simulink model "MPCcontrolledSpacecraft_plant_gnss_kalman_decision"  (R2025b)
settings: Solver=ode113  StartTime=0.0  StopTime=tf  FixedStep=1*60*60  RelTol=1e-8  AbsTol=1e-8
InitFcn:
  | %--- AUTO-INSERTED BY setup_instrument_decision (do not edit by hand)
  | if exist('load_gnss_quality_signals', 'file') == 2
  |     load_gnss_quality_signals('cov_perturb_POS_s6a_Y24D011_fixed.dat');
  | end
  | %--- END AUTO-INSERTED
values from neighbouring files (symbols this model uses):
  area = 15    [Script_Concurso_Spacecraft_batch.m]
  gnss_sample_time = gnssSensor.sample_time    [Script_Concurso_Spacecraft_batch.m]
  h = norm(h_vec)    [Script_Concurso_Spacecraft_batch.m]
  initMass = m_sat    (= 10000)    [Script_Concurso_Spacecraft_batch.m]
  lamda_init = 1    [Script_Concurso_Spacecraft_batch.m]
  m = 3    [Script_Concurso_Spacecraft_batch.m]
  ref = 1.3    [Script_Concurso_Spacecraft_batch.m]
  s = [sigma_x,sigma_x,sigma_x,sigma_v,sigma_v,sigma_v]    [Script_Concurso_Spacecraft_batch.m]
  Ts = 1    [Script_Concurso_Spacecraft_batch.m]
  var_alt = sigma_alt^2    (= 2500)    [Script_Concurso_Spacecraft_batch.m]
  var_IMU = 0.01    [Script_Concurso_Spacecraft_batch.m]
  var_pos = sigma_pos^2    (= 10000)    [Script_Concurso_Spacecraft_batch.m]
undefined symbols (not defined in the file or in its folder): endDate, thrustingThreshold
libraries: simulink x6, vrlib x2, sharedTrackingLibrary x1, aerolibsatdyn x1, aerolibutil x1
settings Model: SimulationMode=accelerator  Creator=benit  LastModifiedBy=benit
settings DebuggingCC: UnderSpecifiedDimensionMsg=warning

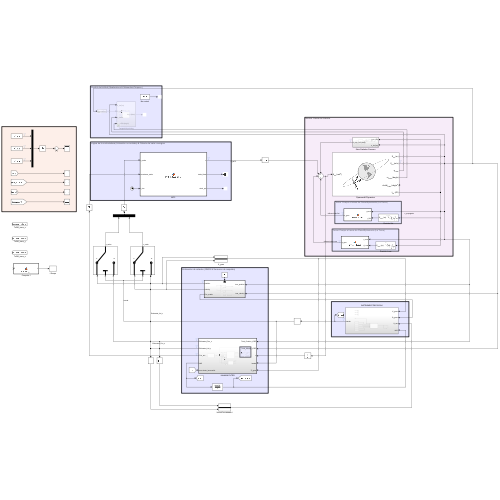
[thumbnail: Simulink's stored preview of the top-level diagram]
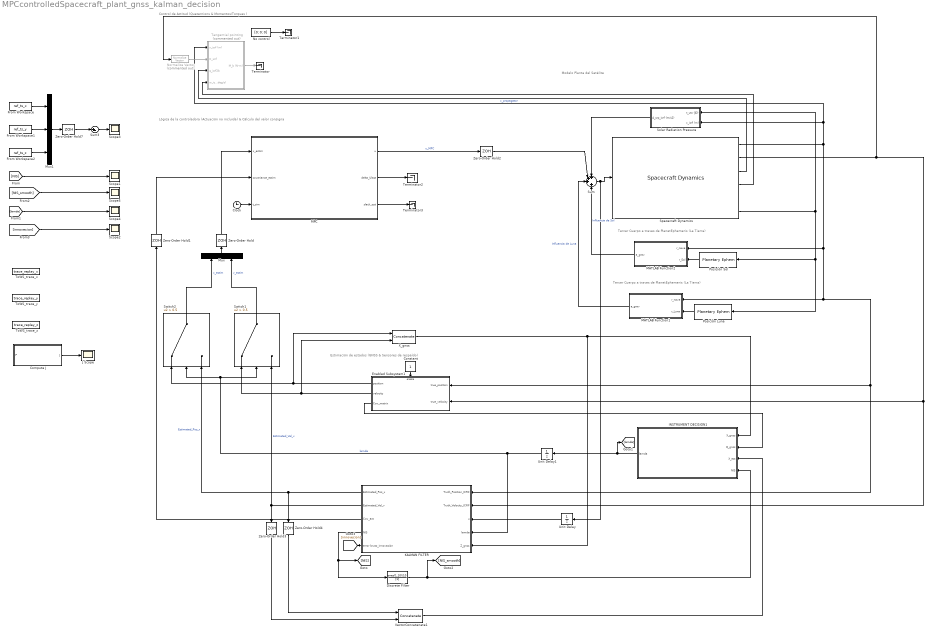
== system MPCcontrolledSpacecraft_plant_gnss_kalman_decision ==
  note: Control de Actitud (Quaternions & Momentos/Torques )
  note: Lógica de la controladora (Actuación no incluida) & Cálculo del valor consigna
  note: Estimación de estados (GNSS & Sensores de respaldo)
  note: Modelo Planta del Satélite
  note: Tercer Cuerpo a traves de PlanetEphemeris (La Tierra)
  note: Tercer Cuerpo a traves de PlanetEphemeris (La Tierra)
  Clock : Clock
      settings: Decimation=h
  Compute J : MATLAB Function  TreatAsAtomicUnit=on
  Constant : Constant
  Discrete Filter : DiscreteFilter  Numerator=ones(1,10)/10  Denominator=[1]
  Enabled Subsystem1 : Subsystem  Description=|  TreatAsAtomicUnit=on
      | "GNSS ON"
      | 
      | Aquí va a ir las medidas del vector de estados utilizando GNSS. 
      | 
      | Se tendrá que añadir todo el sistema de ruido blanco del sensor, así como la regresión
      | por medio de mínimos cuadrados (WLSQ)
  From Workspace : FromWorkspace  VariableName=ref_ts_x  SampleTime=1
  From Workspace1 : FromWorkspace  VariableName=ref_ts_y  SampleTime=1
  From Workspace2 : FromWorkspace  VariableName=ref_ts_z  SampleTime=1
  INSTRUMENT DECISION1 : Subsystem
  J Scope : Scope
      settings: ActiveDisplayYMinimum=-61.078405392126143  ActiveDisplayYMaximum=582.31960931045694
  KALMAN FILTER : Subsystem  Description=|  TreatAsAtomicUnit=on
      | "GNSS OFF"
      | 
      | Aquí va a ir las medidas del vector de estados utilizando Backup Sensor. 
      | 
      | Se tendrá que añadir todo el sistema de ruido blanco de los sensor de respaldo, 
      | así como el Filtro de Kalman y la estadística que permita mezclar las distintas medidas 
      | de distinta procedencia.
  MATLAB Function1 : MATLAB Function  TreatAsAtomicUnit=on
  MATLAB Function2 : MATLAB Function  TreatAsAtomicUnit=on
  MPC : MATLAB Function  TreatAsAtomicUnit=on  SystemSampleTime=h
  Mux : Mux  Inputs=2
  Mux1 : Mux  Inputs=3
  No control : Constant  Value=[0; 0; 0]
  Normalize Vector : vrlib/Utilities/Normalize Vector  Commented=on  maxzero=0
  Posición Luna : PlanetaryEphem  units=m,m/s  center=Sun  startDate=startDate2  endDate=endDate*1.02  outputVelocity=off
  Posición Sol : PlanetaryEphem  units=m,m/s  target=Sun  startDate=startDate2  endDate=endDate*1.02  outputVelocity=off
  Scope{1..5} (5 alike) : Scope
      Scope1 settings: ActiveDisplayYMinimum=-148.75157681735678  ActiveDisplayYMaximum=1338.765518425161
      Scope2 settings: ActiveDisplayYMinimum=-421.91395094944164  ActiveDisplayYMaximum=389.67502541979775  DataLoggingVariableName=ScopeData9
      Scope3 settings: ActiveDisplayYMinimum=-16012.819311832352  ActiveDisplayYMaximum=11977.80759284162  DataLoggingVariableName=ScopeData5
      Scope4 settings: ActiveDisplayYMinimum=-0.12499999999999997  ActiveDisplayYMaximum=1.125  DataLoggingVariableName=ScopeData2
      Scope5 settings: ActiveDisplayYMinimum=-29.897403423774861  ActiveDisplayYMaximum=269.07860039987031  DataLoggingVariableName=ScopeData6
  Solar Radiation Pressure : Subsystem
  Spacecraft Dynamics : SpacecraftDynamics  forcesIn=off  momentsIn=off  accelIn=on  startDate=start_date  mass=m_sat  semiMajorAxis=a  eccentricity=ecc  inclination=inc  raan=RAAN  argPeriapsis=w  trueAnomaly=theta  outputAngAccel=on  shDegree=2  ephemerisStartDate=start_date  ephemerisEndDate=start_date
  Sum : Sum  Inputs=+++|+
  Sum3 : Sum  Inputs=|+-
  Switch1 : Switch  Criteria=u2 > Threshold  Threshold=0.5  SaturateOnIntegerOverflow=off  InputSameDT=off
  Switch2 : Switch  Criteria=u2 > Threshold  Threshold=0.5  SaturateOnIntegerOverflow=off  InputSameDT=off
  Tangential pointing : Subsystem  Commented=on
  Terminator{,1..3} (4 alike) : Terminator
  ToWS_trace_x : ToWorkspace  VariableName=trace_replay_x  SampleTime=-1
  ToWS_trace_y : ToWorkspace  VariableName=trace_replay_y  SampleTime=-1
  ToWS_trace_z : ToWorkspace  VariableName=trace_replay_z  SampleTime=-1
  Unit Delay : UnitDelay  InitialCondition=[0; 0; 0]  SampleTime=Ts  HasFrameUpgradeWarning=on
  Unit Delay1 : UnitDelay  InitialCondition=lamda_init  SampleTime=Ts  HasFrameUpgradeWarning=on
  VectorConcatenate1 : Concatenate
  X_gnss : Concatenate
  Zero-Order Hold{,1..4,7} (6 alike) : ZeroOrderHold  SampleTime=h
  wires:
  Spacecraft Dynamics/1 -> Tangential pointing/1(x_icrf (m)), Solar Radiation Pressure/2(x_icrf (m)), Enabled Subsystem1/1(true_position), KALMAN FILTER/1(Truth_Position_ICRF), MATLAB Function1/1(r_nave), MATLAB Function2/1(r_nave)  "x_propagator"
  Spacecraft Dynamics/6 -> Solar Radiation Pressure/1(t_utc (JD)), Posición Luna/1, Posición Sol/1
  Posición Sol/1 -> MATLAB Function2/2(r_Sol)
  Posición Luna/1 -> MATLAB Function1/2(r_Luna)
  Unit Delay1/1 -> Switch2/2, Switch1/2, KALMAN FILTER/4(lamda)  "lamda"
  Spacecraft Dynamics/2 -> KALMAN FILTER/2(Truth_Velocity_ICRF), Enabled Subsystem1/2(true_velocity), Normalize Vector/1
  Enabled Subsystem1/1(position) -> Switch2/1, X_gnss/1
  KALMAN FILTER/1(Estimated_Pos_x) -> Switch2/3, Zero-Order Hold4/1  "Estimated_Pos_x"
  Spacecraft Dynamics/4 -> Tangential pointing/4(w_icrf2b (deg/s))
  Spacecraft Dynamics/3 -> Tangential pointing/3(q_icrf2b)
  Normalize Vector/1 -> Tangential pointing/2(C_icrf)
  Tangential pointing/1(M_b (N-m)) -> Terminator/1
  No control/1 -> Terminator1/1
  Enabled Subsystem1/2(velocity) -> Switch1/1, X_gnss/2
  KALMAN FILTER/2(Estimated_Vel_v) -> Switch1/3, Zero-Order Hold3/1  "Estimated_Vel_v"
  Solar Radiation Pressure/1(A_srp_icrf (m/s2)) -> Sum/1
  MATLAB Function2/1(a_grav) -> Sum/4  "Influencia de Sol"
  MATLAB Function1/1(a_grav) -> Sum/3  "Influencia de Luna"
  Sum/1 -> Spacecraft Dynamics/1, Unit Delay/1
  KALMAN FILTER/3(Cov_act) -> Zero-Order Hold1/1
  Unit Delay/1 -> KALMAN FILTER/3(u)
  Mux/1 -> Zero-Order Hold/1
  MPC/1(u) -> Zero-Order Hold2/1  "u_MPC"
  MPC/2(delta_Ulast) -> Terminator2/1
  MPC/3(slack_opt) -> Terminator3/1
  Zero-Order Hold/1 -> MPC/1(x_estim)
  Zero-Order Hold1/1 -> MPC/2(covariance_estim)
  Zero-Order Hold2/1 -> Sum/2
  Clock/1 -> MPC/3(t_sim)
  X_gnss/1 -> KALMAN FILTER/5(Z_gnss), INSTRUMENT DECISION1/1(X_gnss)
  Enabled Subsystem1/3(Cov_matrix) -> INSTRUMENT DECISION1/2(Q_gnss)
  VectorConcatenate1/1 -> INSTRUMENT DECISION1/3(X_est)
  Zero-Order Hold3/1 -> VectorConcatenate1/2
  Zero-Order Hold4/1 -> VectorConcatenate1/1
  Switch2/1 -> Mux/1  "x_estim"
  Switch1/1 -> Mux/2  "v_estim"
  Constant/1 -> Enabled Subsystem1/Enable
  Compute J/1(J) -> J Scope/1
  From Workspace1/1 -> Mux1/2
  From Workspace/1 -> Mux1/1
  From Workspace2/1 -> Mux1/3
  Mux1/1 -> Zero-Order Hold7/1
  Sum3/1 -> Scope3/1
  KALMAN FILTER/4(NIS) -> [NIS], Discrete Filter/1
  [NIS] -> Scope1/1
  [lamda] -> Scope4/1
  Zero-Order Hold7/1 -> Sum3/1
  Discrete Filter/1 -> [NIS_smooth], INSTRUMENT DECISION1/4(NIS)
  [NIS_smooth] -> Scope5/1
  INSTRUMENT DECISION1/1(lamda) -> Unit Delay1/1, [lamda]
  KALMAN FILTER/5(error bruto_innovación) -> [innovecion]
  [innovecion] -> Scope2/1

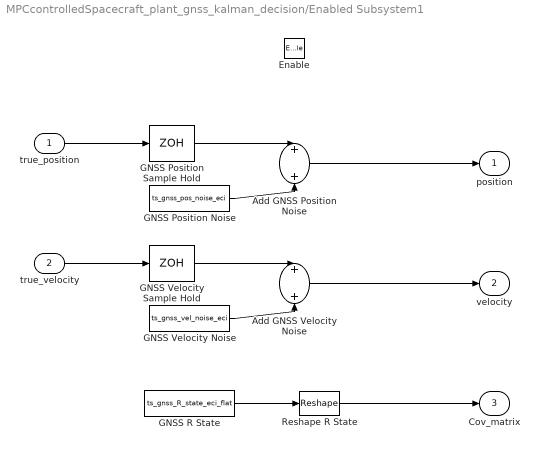
== system MPCcontrolledSpacecraft_plant_gnss_kalman_decision/Enabled Subsystem1 ==
  true_position : Inport
  true_velocity : Inport  Port=2
  Enable : EnablePort
  Add GNSS Position Noise : Sum
  Add GNSS Velocity Noise : Sum
  GNSS Position Noise : FromWorkspace  VariableName=ts_gnss_pos_noise_eci  SampleTime=Ts
  GNSS Position Sample Hold : ZeroOrderHold  SampleTime=gnss_sample_time
  GNSS R State : FromWorkspace  VariableName=ts_gnss_R_state_eci_flat  SampleTime=Ts
  GNSS Velocity Noise : FromWorkspace  VariableName=ts_gnss_vel_noise_eci  SampleTime=Ts
  GNSS Velocity Sample Hold : ZeroOrderHold  SampleTime=gnss_sample_time
  Reshape R State : Reshape  OutputDimensionality=Customize  OutputDimensions=[6 6]
  position : Outport  InitialOutput=zeros(3,1)
  velocity : Outport  Port=2  InitialOutput=zeros(3,1)
  Cov_matrix : Outport  Port=3  InitialOutput=zeros(6,6)
  wires:
  true_position/1 -> GNSS Position Sample Hold/1
  GNSS Position Sample Hold/1 -> Add GNSS Position Noise/1
  GNSS Position Noise/1 -> Add GNSS Position Noise/2
  Add GNSS Position Noise/1 -> position/1
  true_velocity/1 -> GNSS Velocity Sample Hold/1
  GNSS Velocity Sample Hold/1 -> Add GNSS Velocity Noise/1
  GNSS Velocity Noise/1 -> Add GNSS Velocity Noise/2
  Add GNSS Velocity Noise/1 -> velocity/1
  GNSS R State/1 -> Reshape R State/1
  Reshape R State/1 -> Cov_matrix/1

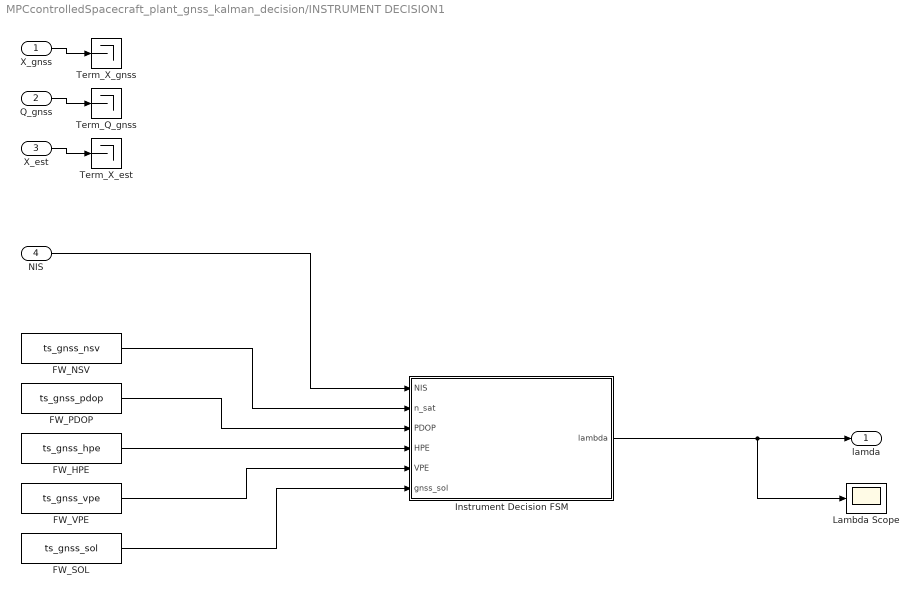
== system MPCcontrolledSpacecraft_plant_gnss_kalman_decision/INSTRUMENT DECISION1 ==
  X_gnss : Inport
  Q_gnss : Inport  Port=2
  X_est : Inport  Port=3
  NIS : Inport  Port=4
  FW_HPE : FromWorkspace  VariableName=ts_gnss_hpe  SampleTime=Ts  Interpolate=off  ZeroCross=off  OutputAfterFinalValue=Holding final value
  FW_NSV : FromWorkspace  VariableName=ts_gnss_nsv  SampleTime=Ts  Interpolate=off  ZeroCross=off  OutputAfterFinalValue=Holding final value
  FW_PDOP : FromWorkspace  VariableName=ts_gnss_pdop  SampleTime=Ts  Interpolate=off  ZeroCross=off  OutputAfterFinalValue=Holding final value
  FW_SOL : FromWorkspace  VariableName=ts_gnss_sol  SampleTime=Ts  Interpolate=off  ZeroCross=off  OutputAfterFinalValue=Holding final value
  FW_VPE : FromWorkspace  VariableName=ts_gnss_vpe  SampleTime=Ts  Interpolate=off  ZeroCross=off  OutputAfterFinalValue=Holding final value
  Instrument Decision FSM : MATLAB Function  TreatAsAtomicUnit=on
  Lambda Scope : Scope
      settings: ActiveDisplayYMinimum=-0.12499999999999997  ActiveDisplayYMaximum=1.125
  Term_Q_gnss : Terminator
  Term_X_est : Terminator
  Term_X_gnss : Terminator
  lamda : Outport
  wires:
  NIS/1 -> Instrument Decision FSM/1(NIS)
  FW_NSV/1 -> Instrument Decision FSM/2(n_sat)
  FW_PDOP/1 -> Instrument Decision FSM/3(PDOP)
  FW_HPE/1 -> Instrument Decision FSM/4(HPE)
  FW_VPE/1 -> Instrument Decision FSM/5(VPE)
  FW_SOL/1 -> Instrument Decision FSM/6(gnss_sol)
  X_gnss/1 -> Term_X_gnss/1
  Q_gnss/1 -> Term_Q_gnss/1
  X_est/1 -> Term_X_est/1
  Instrument Decision FSM/1(lambda) -> lamda/1, Lambda Scope/1

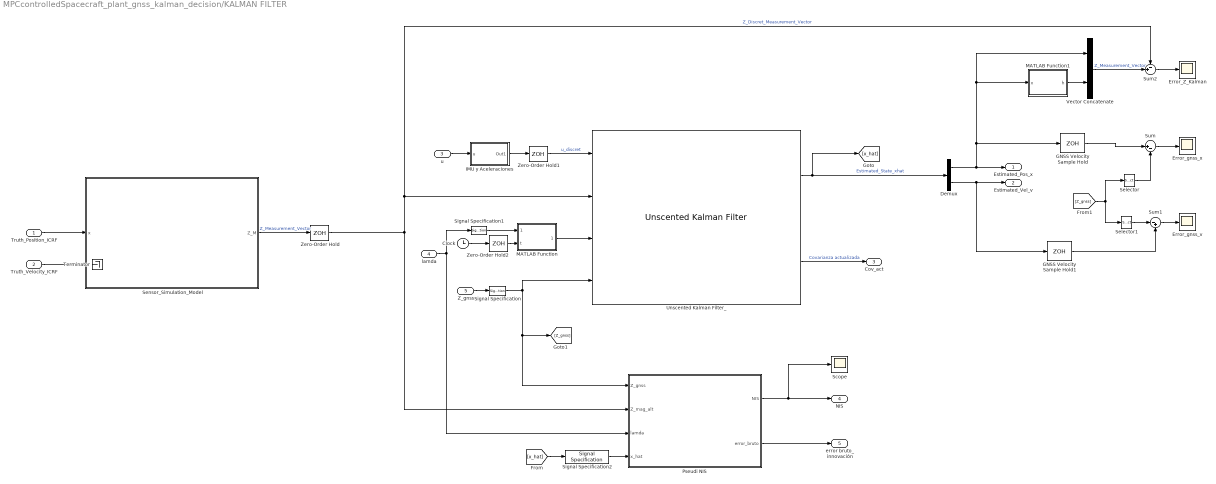
== system MPCcontrolledSpacecraft_plant_gnss_kalman_decision/KALMAN FILTER ==
  Truth_Position_ICRF : Inport
  Truth_Velocity_ICRF : Inport  Port=2
  u : Inport  Port=3  PortDimensions=[3 1]
  lamda : Inport  Port=4
  Z_gnss : Inport  Port=5
  Clock : Clock
  Demux : Demux  Outputs=2
  Error_Z_Kalman : Scope
      settings: ActiveDisplayYMinimum=-488.49081630726869  ActiveDisplayYMaximum=454.68629612577206  DataLoggingVariableName=ScopeData4
  Error_gnss_v : Scope
      settings: ActiveDisplayYMinimum=-3.007134468189463  ActiveDisplayYMaximum=2.2874556586182848  DataLoggingVariableName=ScopeData8
  Error_gnss_x : Scope
      settings: ActiveDisplayYMinimum=-75.440852466621436  ActiveDisplayYMaximum=50.927813746617176  DataLoggingVariableName=ScopeData7
  GNSS Velocity Sample Hold : ZeroOrderHold  SampleTime=gnss_sample_time
  GNSS Velocity Sample Hold1 : ZeroOrderHold  SampleTime=gnss_sample_time
  IMU y Aceleraciones : Subsystem
  MATLAB Function : MATLAB Function  TreatAsAtomicUnit=on
  MATLAB Function1 : MATLAB Function  TreatAsAtomicUnit=on
  Pseudi NIS : MATLAB Function  TreatAsAtomicUnit=on
  Scope : Scope
      settings: ActiveDisplayYMinimum=-1.0362684351466058E+6  ActiveDisplayYMaximum=9.3264159202136155E+6  DataLoggingVariableName=ScopeData3
  Selector : Selector  InputPortWidth=6  IndexOptions=Index vector (dialog)  Indices=[1 2 3]  OutputSizes=1
  Selector1 : Selector  InputPortWidth=6  IndexOptions=Index vector (dialog)  Indices=[4 5 6]  OutputSizes=1
  Sensor_Simulation_Model : Subsystem
  Signal Specification : SignalSpecification  OutDataTypeStr=double  Dimensions=[6, 1]
  Signal Specification1 : SignalSpecification  OutDataTypeStr=boolean  Dimensions=1
  Signal Specification2 : SignalSpecification  Dimensions=[6, 1]
  Sum : Sum  Inputs=|+-
  Sum1 : Sum  Inputs=|-+
  Sum2 : Sum  Inputs=-+|
  Terminator : Terminator
  Unscented Kalman Filter_ : sharedTrackingLibrary/Unscented Kalman Filter  StateTransitionFcn=myStateTransitionFcn  HasAdditiveProcessNoise=Additive  ProcessNoise=Q_matrix  HasTimeVaryingProcessNoise=off  HasStateTransitionFcnExtraArgument=1  InitialState=x0_kalman  InitialStateCovariance=P0_kalman  Alpha=1e-3  Beta=2  Kappa=0  MeasurementFcn1=myMeasurementFcn  HasMeasurementEnablePort1=off  HasAdditiveMeasurementNoise1=Additive  MeasurementNoise1=R_matrix  HasTimeVaryingMeasurementNoise1=off  HasMeasurementFcnExtraArgument1=0  HasMeasurementWrapping1=off  MeasurementFcn2=medida_gnss_fcn  HasMeasurementEnablePort2=on  HasAdditiveMeasurementNoise2=Additive  MeasurementNoise2=R_gnss  HasTimeVaryingMeasurementNoise2=off  HasMeasurementFcnExtraArgument2=0  HasMeasurementWrapping2=off  MeasurementFcn3=myMeasurementFcn  HasMeasurementEnablePort3=off  HasAdditiveMeasurementNoise3=Additive  MeasurementNoise3=1  HasTimeVaryingMeasurementNoise3=off  HasMeasurementFcnExtraArgument3=0  HasMeasurementWrapping3=off  MeasurementFcn4=myMeasurementFcn  HasMeasurementEnablePort4=off  HasAdditiveMeasurementNoise4=Additive  MeasurementNoise4=1  HasTimeVaryingMeasurementNoise4=off  HasMeasurementFcnExtraArgument4=0  HasMeasurementWrapping4=off  MeasurementFcn5=myMeasurementFcn  HasMeasurementEnablePort5=off  HasAdditiveMeasurementNoise5=Additive  MeasurementNoise5=1  HasTimeVaryingMeasurementNoise5=off  HasMeasurementFcnExtraArgument5=0  HasMeasurementWrapping5=off  EnableMultirate=off  StateTransitionFcnSampleTime=1  MeasurementFcn1SampleTime=1  MeasurementFcn2SampleTime=1  MeasurementFcn3SampleTime=1  MeasurementFcn4SampleTime=1  MeasurementFcn5SampleTime=1  UseCurrentEstimator=on  OutputStateCovariance=on  DataType=double  SampleTime=Ts  NumberOfMeasurements=2
      settings: LibrarySourceBlock=cstblocks/State Estimation/Unscented Kalman Filter
  Vector Concatenate : Concatenate
  Zero-Order Hold : ZeroOrderHold  SampleTime=Ts
  Zero-Order Hold1 : ZeroOrderHold  SampleTime=Ts
  Zero-Order Hold2 : ZeroOrderHold  SampleTime=Ts
  Estimated_Pos_x : Outport
  Estimated_Vel_v : Outport  Port=2
  Cov_act : Outport  Port=3
  NIS : Outport  Port=4
  error bruto_innovación : Outport  Port=5
  wires:
  Truth_Velocity_ICRF/1 -> Terminator/1
  Unscented Kalman Filter_/1 -> Demux/1, [x_hat]  "Estimated_State_xhat"
  Unscented Kalman Filter_/2 -> Cov_act/1  "Covarianza actualizada"
  Truth_Position_ICRF/1 -> Sensor_Simulation_Model/1(x)
  Demux/2 -> GNSS Velocity Sample Hold1/1, Estimated_Vel_v/1
  Sensor_Simulation_Model/1(Z_M) -> Zero-Order Hold/1  "Z_Measurement_Vector"
  Zero-Order Hold/1 -> Unscented Kalman Filter_/2, Sum2/1, Pseudi NIS/2(Z_mag_alt)  "Z_Discret_Measurement_Vector"
  Zero-Order Hold1/1 -> Unscented Kalman Filter_/1  "u_discret"
  u/1 -> IMU y Aceleraciones/1(u)
  IMU y Aceleraciones/1(Out1) -> Zero-Order Hold1/1
  Z_gnss/1 -> Signal Specification/1
  Signal Specification/1 -> Pseudi NIS/1(Z_gnss), [Z_gnss], Unscented Kalman Filter_/4
  Selector/1 -> Sum/2
  [Z_gnss] -> Selector1/1, Selector/1
  Sum/1 -> Error_gnss_x/1
  Selector1/1 -> Sum1/1
  Sum1/1 -> Error_gnss_v/1
  MATLAB Function/1(enable_gnss) -> Unscented Kalman Filter_/3
  Demux/1 -> Estimated_Pos_x/1, GNSS Velocity Sample Hold/1, MATLAB Function1/1(x), Vector Concatenate/1
  lamda/1 -> Pseudi NIS/3(lamda), Signal Specification1/1
  Clock/1 -> Zero-Order Hold2/1
  Zero-Order Hold2/1 -> MATLAB Function/2(t)
  Signal Specification1/1 -> MATLAB Function/1(lambda)
  GNSS Velocity Sample Hold1/1 -> Sum1/2
  GNSS Velocity Sample Hold/1 -> Sum/1
  [x_hat] -> Signal Specification2/1
  Signal Specification2/1 -> Pseudi NIS/4(x_hat)
  Sum2/1 -> Error_Z_Kalman/1
  MATLAB Function1/1(h) -> Vector Concatenate/2
  Vector Concatenate/1 -> Sum2/2  "Z_Measurement_Vector"
  Pseudi NIS/1(NIS) -> Scope/1, NIS/1
  Pseudi NIS/2(error_bruto) -> error bruto_innovación/1

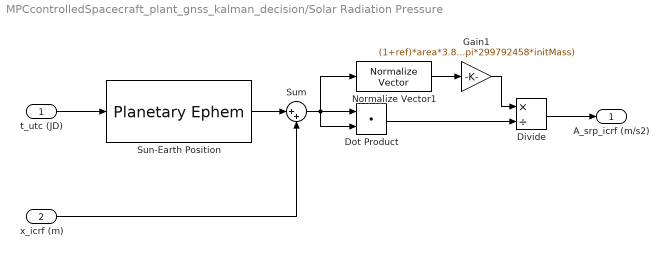
== system MPCcontrolledSpacecraft_plant_gnss_kalman_decision/Solar Radiation Pressure ==
  t_utc (JD) : Inport
  x_icrf (m) : Inport  Port=2
  Divide : Product  Inputs=*/
  Dot Product : DotProduct  OutDataTypeStr=Inherit: Inherit via internal rule
  Gain1 : Gain  Gain=(1+ref)*area*3.852e26/(4*pi*299792458*initMass)
  Normalize Vector1 : vrlib/Utilities/Normalize Vector  maxzero=0
  Sum : Sum  Inputs=|++
  Sun-Earth Position : PlanetaryEphem  units=m,m/s  center=Sun  target=Earth  outputVelocity=off
  A_srp_icrf (m/s2) : Outport
  wires:
  Normalize Vector1/1 -> Gain1/1
  Gain1/1 -> Divide/1
  Dot Product/1 -> Divide/2
  Divide/1 -> A_srp_icrf (m/s2)/1
  t_utc (JD)/1 -> Sun-Earth Position/1
  Sun-Earth Position/1 -> Sum/1
  Sum/1 -> Dot Product/1, Normalize Vector1/1, Dot Product/2
  x_icrf (m)/1 -> Sum/2

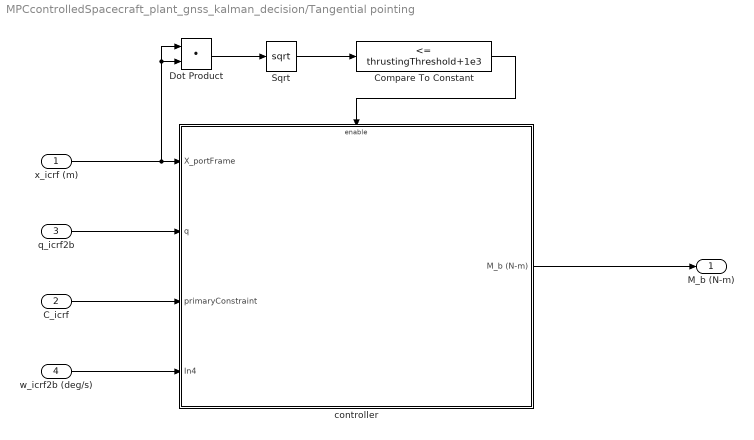
== system MPCcontrolledSpacecraft_plant_gnss_kalman_decision/Tangential pointing ==
  x_icrf (m) : Inport
  C_icrf : Inport  Port=2
  q_icrf2b : Inport  Port=3
  w_icrf2b (deg/s) : Inport  Port=4
  Compare To Constant : simulink/Logic and Bit Operations/Compare To Constant  relop=<=  const=thrustingThreshold+1e3  OutDataTypeStr=boolean
  Dot Product : DotProduct  OutDataTypeStr=Inherit: Inherit via internal rule
  Sqrt : Sqrt
  controller : Subsystem
  M_b (N-m) : Outport
  wires:
  q_icrf2b/1 -> controller/2(q)
  C_icrf/1 -> controller/3(primaryConstraint)
  w_icrf2b (deg/s)/1 -> controller/4(In4)
  controller/1(M_b (N-m)) -> M_b (N-m)/1
  Dot Product/1 -> Sqrt/1
  Sqrt/1 -> Compare To Constant/1
  x_icrf (m)/1 -> Dot Product/1, Dot Product/2, controller/1(X_portFrame)
  Compare To Constant/1 -> controller/Enable

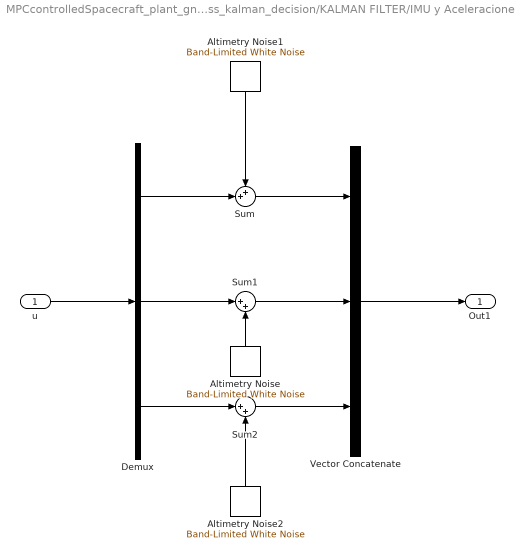
== system MPCcontrolledSpacecraft_plant_gnss_kalman_decision/KALMAN FILTER/IMU y Aceleraciones ==
  u : Inport  PortDimensions=[3 1]
  Altimetry Noise : simulink/Sources/Band-Limited White Noise  Cov=var_IMU* Ts  Ts=Ts  seed=[23341]
  Altimetry Noise1 : simulink/Sources/Band-Limited White Noise  Cov=var_IMU* Ts  Ts=Ts  seed=[23341]
  Altimetry Noise2 : simulink/Sources/Band-Limited White Noise  Cov=var_IMU* Ts  Ts=Ts  seed=[23341]
  Demux : Demux  Outputs=3
  Sum : Sum  Inputs=++|
  Sum1 : Sum  Inputs=|++
  Sum2 : Sum  Inputs=|++
  Vector Concatenate : Concatenate  NumInputs=3
  Out1 : Outport
  wires:
  Vector Concatenate/1 -> Out1/1
  u/1 -> Demux/1
  Demux/1 -> Sum/2
  Altimetry Noise1/1 -> Sum/1
  Demux/3 -> Sum2/1
  Altimetry Noise2/1 -> Sum2/2
  Demux/2 -> Sum1/1
  Altimetry Noise/1 -> Sum1/2
  Sum/1 -> Vector Concatenate/1
  Sum2/1 -> Vector Concatenate/3
  Sum1/1 -> Vector Concatenate/2

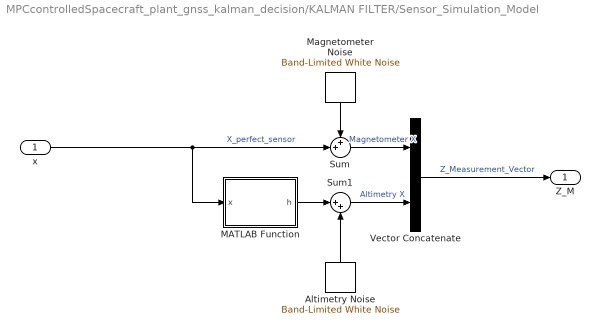
== system MPCcontrolledSpacecraft_plant_gnss_kalman_decision/KALMAN FILTER/Sensor_Simulation_Model ==
  x : Inport
  Altimetry Noise : simulink/Sources/Band-Limited White Noise  Cov=var_alt* Ts  Ts=Ts  seed=[23341]
  MATLAB Function : MATLAB Function  TreatAsAtomicUnit=on
  Magnetometer Noise : simulink/Sources/Band-Limited White Noise  Cov=var_pos * Ts  Ts=Ts  seed=[23341]
  Sum : Sum  Inputs=++|
  Sum1 : Sum  Inputs=|++
  Vector Concatenate : Concatenate
  Z_M : Outport
  wires:
  x/1 -> MATLAB Function/1(x), Sum/2  "X_perfect_sensor"
  Altimetry Noise/1 -> Sum1/2
  Sum/1 -> Vector Concatenate/1  "Magnetometer X"
  MATLAB Function/1(h) -> Sum1/1
  Magnetometer Noise/1 -> Sum/1
  Sum1/1 -> Vector Concatenate/2  "Altimetry X"
  Vector Concatenate/1 -> Z_M/1  "Z_Measurement_Vector"

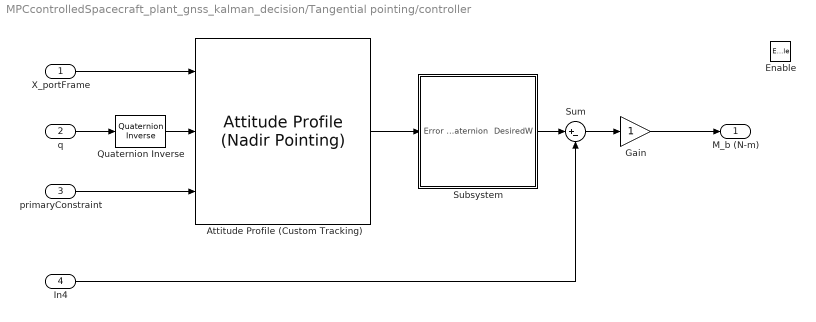
== system MPCcontrolledSpacecraft_plant_gnss_kalman_decision/Tangential pointing/controller ==
  X_portFrame : Inport
  q : Inport  Port=2
  primaryConstraint : Inport  Port=3
  In4 : Inport  Port=4
  Enable : EnablePort
  Attitude Profile (Custom Tracking) : aerolibsatdyn/Attitude Profile (Nadir Pointing)  outputError=on  outputFinalAttitude=off  portFrame=ICRF  pointingMode=Custom  celestialTarget=Sun  tunablePointing=off  primaryAlignmentSrc=Dialog  primaryAlignment=[1 0 0]  secondaryAlignmentSrc=Dialog  secondaryAlignment=[0 0 1]  constraintFrame=ICRF  primaryConstraintSrc=Port  primaryConstraint=[1 0 0]  secondaryConstraintSrc=Dialog  secondaryConstraint=[0 0 1]
      settings: LibrarySourceBlock=|
      | aerolibsatdyn/Attitude Profile
      | (Sun Tracking)
  Gain : Gain
  Quaternion Inverse : aerolibutil/Quaternion Inverse
  Subsystem : Subsystem
  Sum : Sum  Inputs=|+-
  M_b (N-m) : Outport
  wires:
  X_portFrame/1 -> Attitude Profile (Custom Tracking)/1
  Sum/1 -> Gain/1
  primaryConstraint/1 -> Attitude Profile (Custom Tracking)/3
  Quaternion Inverse/1 -> Attitude Profile (Custom Tracking)/2
  Attitude Profile (Custom Tracking)/1 -> Subsystem/1(Error quaternion)
  Gain/1 -> M_b (N-m)/1
  Subsystem/1(DesiredW) -> Sum/1
  In4/1 -> Sum/2
  q/1 -> Quaternion Inverse/1

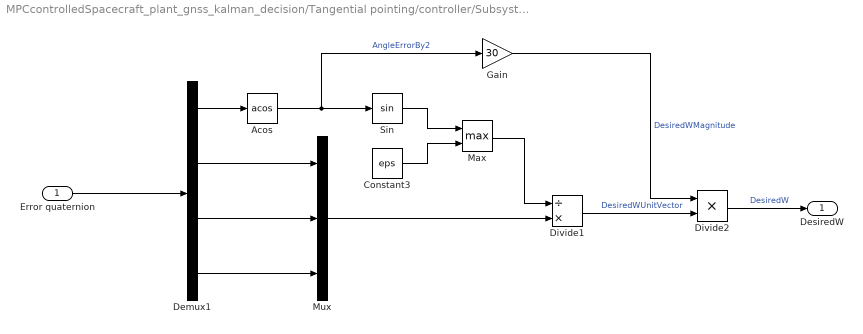
== system MPCcontrolledSpacecraft_plant_gnss_kalman_decision/Tangential pointing/controller/Subsystem ==
  Error quaternion : Inport
  Acos : Trigonometry  Operator=acos
  Constant3 : Constant  Value=eps
  Demux1 : Demux
  Divide1 : Product  Inputs=/*
  Divide2 : Product  Inputs=**
  Gain : Gain  Gain=30
  Max : MinMax  Function=max  Inputs=2
  Mux : Mux  Inputs=3
  Sin : Trigonometry
  DesiredW : Outport
  wires:
  Error quaternion/1 -> Demux1/1
  Gain/1 -> Divide2/1  "DesiredWMagnitude"
  Demux1/2 -> Mux/1
  Demux1/1 -> Acos/1
  Acos/1 -> Sin/1, Gain/1  "AngleErrorBy2"
  Mux/1 -> Divide1/2
  Divide2/1 -> DesiredW/1  "DesiredW"
  Constant3/1 -> Max/2
  Demux1/3 -> Mux/2
  Max/1 -> Divide1/1
  Demux1/4 -> Mux/3
  Sin/1 -> Max/1
  Divide1/1 -> Divide2/2  "DesiredWUnitVector"

== matlab function MPCcontrolledSpacecraft_plant_gnss_kalman_decision/MATLAB Function1 ==
  data: r_nave input; a_grav output; r_Luna input
function a_grav = gravedadLuna(r_nave, r_Luna)
%#codegen

% Constante gravitacional de Marte
mu_Luna = 4.90e12; % [m^3/s^2]

% Vector relativo
r_rel = r_nave - r_Luna;

% Magnitud de la distancia
dist = norm(r_rel);

% Aceleración gravitatoria
a_grav = (-mu_Luna / dist^3) * r_rel;

end

== matlab function MPCcontrolledSpacecraft_plant_gnss_kalman_decision/KALMAN FILTER/Sensor_Simulation_Model/MATLAB Function ==
  data: x input; h output
function h = altimetry(x)
% Cálculo de la distancia radial
R_Tierra= 6378137.0;       % Radio ecuatorial [m]
h=sqrt((x(1)^2)+(x(2)^2)+(x(3)^2))-R_Tierra;

== matlab function MPCcontrolledSpacecraft_plant_gnss_kalman_decision/MATLAB Function2 ==
  data: r_nave input; a_grav output; r_Sol input
function a_grav = gravedadSol(r_nave, r_Sol)
%#codegen

% Constante gravitacional de Marte
mu_sol = 1.327e20; % [m^3/s^2]

% Vector relativo
r_rel = r_nave - r_Sol;

% Magnitud de la distancia
dist = norm(r_rel);

% Aceleración gravitatoria
a_grav = (-mu_sol / dist^3) * r_rel;

end

== matlab function MPCcontrolledSpacecraft_plant_gnss_kalman_decision/Compute J ==
  data: P input; J output
function J = compute_J(P)
%#codegen
% J = trace(S_inv * P * S_T_inv) with sigma_x=10, sigma_v=1
sigma_x=10;
sigma_v=1;
S_inv   = diag([1/sigma_x,1/sigma_x,1/sigma_x,1/sigma_v,1/sigma_v,1/sigma_v]);
S_T_inv = diag([1/sigma_x,1/sigma_x,1/sigma_x,1/sigma_v,1/sigma_v,1/sigma_v]);
n = numel(P);
if n == 36
    Pm = reshape(P,6,6);
elseif n == 6
    Pm = diag(P(:));
elseif n == 1
    J = double(P);
    return;
else
    Pm = reshape(P,6,6);  % best effort
end
J = trace(S_inv * Pm * S_T_inv);
end

== matlab function MPCcontrolledSpacecraft_plant_gnss_kalman_decision/MPC ==
  data: x_estim input; covariance_estim input; t_sim input; u output; delta_Ulast output; slack_opt output
function [u, delta_Ulast, slack_opt] = MPC_INOAS_block(x_estim, covariance_estim, t_sim)

%#codegen
coder.extrinsic('MPC_INOAS');

u = zeros(3,1);
delta_Ulast = zeros(150,1);
slack_opt = zeros(50,1);

[u_tmp, delta_tmp, slack_tmp] = MPC_INOAS(x_estim, covariance_estim, t_sim);

u = u_tmp;
delta_Ulast = delta_tmp;
slack_opt = slack_tmp;

end

== matlab function MPCcontrolledSpacecraft_plant_gnss_kalman_decision/KALMAN FILTER/Pseudi NIS ==
  data: Z_gnss input size=[6, 1]; Z_mag_alt input; lamda input; NIS output; x_hat input size=[6, 1]; error_bruto output
function [NIS, error_bruto] = compute_NIS(Z_gnss, Z_mag_alt, lamda, x_hat)
%#codegen

    persistent Z_gnss_prev x_hat_held
    if isempty(Z_gnss_prev)
        Z_gnss_prev = zeros(6,1);
        x_hat_held = zeros(6,1);
    end
    
    % --- ZOH POR SOFTWARE MEJORADO ---
    % Ignoramos los temblores del ruido (< 100m)
    % Solo hacemos foto cuando el GNSS pega el salto real de la órbita (> 1000m)
    if sum(abs(Z_gnss(1:3) - Z_gnss_prev(1:3))) > 1000
        x_hat_held = x_hat;
        Z_gnss_prev = Z_gnss;
    end

    R_tierra = 6378137.0; 

    if lamda == 1
        % --- MODO 1: GNSS ---
        sigma_pos_gnss = 5;   
        sigma_vel_gnss = 0.1; 
        
        R_inv = diag([1/sigma_pos_gnss^2, 1/sigma_pos_gnss^2, 1/sigma_pos_gnss^2, ...
                      1/sigma_vel_gnss^2, 1/sigma_vel_gnss^2, 1/sigma_vel_gnss^2]);
                  
        Z_pred = x_hat_held; 
        y = Z_gnss - Z_pred;
        
    else
        % --- MODO 0: MAGNETÓMETRO + ALTÍMETRO ---
        sigma_mag = 300; 
        sigma_alt = 50;  
        
        R_inv = diag([1/sigma_mag^2, 1/sigma_mag^2, 1/sigma_mag^2, 1/sigma_alt^2]);
        
        pos_pred = [x_hat(1); x_hat(2); x_hat(3)];
        r_norm = norm(pos_pred);
        alt_pred = r_norm - R_tierra;
        
        Z_pred = [pos_pred(1); pos_pred(2); pos_pred(3); alt_pred];
        
        y = Z_mag_alt - Z_pred;
    end
    
    y_col = y(:); 
    NIS = y_col' * R_inv * y_col;
    
    % --- EL ESCÁNER ---
    error_bruto = zeros(6,1);
    for i = 1:length(y_col)
        error_bruto(i) = y_col(i);
    end
end

== matlab function MPCcontrolledSpacecraft_plant_gnss_kalman_decision/KALMAN FILTER/MATLAB Function ==
  data: lambda input; enable_gnss output; t input
function enable_gnss = gatillo_gnss(lambda, t)
    %#codegen
    % Frecuencia del GNSS en segundos (cámbialo a 3 si tu ZOH es de 3s)
    gnss_rate = 3; 
    
    % Comprobamos si estamos en un segundo exacto múltiplo de 10
    % (Usamos round para evitar errores de precisión de los decimales)
    is_new_data = mod(round(t), gnss_rate) == 0;
    
    % Solo abrimos la puerta si la máquina lo pide Y hay dato fresco
    enable_gnss = lambda && is_new_data;
end

== matlab function MPCcontrolledSpacecraft_plant_gnss_kalman_decision/INSTRUMENT DECISION1/Instrument Decision FSM ==
  data: NIS input; lambda output; n_sat input; PDOP input; HPE input; VPE input; gnss_sol input
function lambda = instrument_decision(NIS, n_sat, PDOP, HPE, VPE, gnss_sol)
% INSTRUMENT_DECISION  State machine: GNSS vs Kalman selector
%   Outputs lambda = 1 (GNSS active)  or  0 (Kalman propagation only).
%
% INPUTS
%   NIS      - Normalized Innovation Squared from auxiliary sensors [scalar]
%   n_sat    - number of GNSS satellites used (NSV)
%   PDOP     - position dilution of precision
%   HPE,VPE  - horizontal / vertical position error [m]
%   gnss_sol - GNSS solution validity flag (1 valid, 0 no-fix)
%
% BEHAVIOUR
%   GNSS   -> KALMAN : timer >= T_gnss_on  (periodic duty cycle)
%                      OR any Table-3.1 emergency condition
%   KALMAN -> GNSS   : timer >= T_kalman_on AND GNSS healthy
%                      OR NIS >= max_NIS AND GNSS healthy
%#codegen
persistent state timer_count;

% --- Parameters ----------------------------------------------------------
T_gnss_on   = 60;   % [s] GNSS ON period before switching to Kalman
T_kalman_on = 60;   % [s] Kalman ON period before returning to GNSS
max_NIS     = 2;   % NIS threshold for forced return to GNSS (aprox 400m error)
n_sat_min   = 4;    % minimum satellites for a valid fix  (Table 3.1)
PDOP_max    = 6;    % PDOP limit                          (Table 3.1)
HPE_max     = 5;    % horizontal position error limit [m] (Table 3.1)
VPE_max     = 5;    % vertical   position error limit [m] (Table 3.1)
Ts          = 1;    % [s] execution sample time of this decision block

GNSS_STATE   = int32(0);
KALMAN_STATE = int32(1);

if isempty(state)
    state       = GNSS_STATE;
    timer_count = int32(0);
end

% --- Table-3.1 emergency conditions -------------------------------------
signal_outage   = (n_sat < n_sat_min) || (gnss_sol < 0.5);
precision_loss  = (HPE > HPE_max)     || (VPE > VPE_max);
geometric_drift = (PDOP > PDOP_max);
emergency       = signal_outage || precision_loss || geometric_drift;

timer_count = timer_count + int32(Ts);

switch state
    case GNSS_STATE
        if emergency
            % Immediate forced switch - GNSS is unusable
            state       = KALMAN_STATE;
            timer_count = int32(0);
        elseif timer_count >= int32(T_gnss_on)
            % Periodic duty-cycle: GNSS has been on long enough
            state       = KALMAN_STATE;
            timer_count = int32(0);
        end
        
    case KALMAN_STATE
        % Real duty-cycle: leave Kalman after its ON window, or earlier if
        % sensor discrepancy (NIS) becomes too large.
        gnss_healthy = ~emergency;
        
        if gnss_healthy && ((timer_count >= int32(T_kalman_on)) || (NIS >= max_NIS))
            state       = GNSS_STATE;
            timer_count = int32(0);
        end
        
    otherwise
        state       = GNSS_STATE;
        timer_count = int32(0);
end

%lambda = double(state == GNSS_STATE);
lambda = logical(state == GNSS_STATE);
end

== matlab function MPCcontrolledSpacecraft_plant_gnss_kalman_decision/KALMAN FILTER/MATLAB Function1 ==
  data: x input; h output
function h = altimetry(x)
% Cálculo de la distancia radial
R_Tierra= 6378137.0;       % Radio ecuatorial [m]
h=sqrt((x(1)^2)+(x(2)^2)+(x(3)^2))-R_Tierra;
